simulink library "FIBlockLib"  (R2021a)
settings: Solver=VariableStepAuto  StartTime=0.0  StopTime=10.0  RelTol=1e-3
settings Model: Creator=flata  LastModifiedBy=DELL
settings SolverCC: AlgebraicLoopSolver=TrustRegion
settings DebuggingCC: SFMachineParentedDataDiag=warning

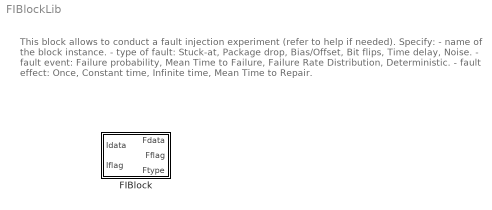
== system FIBlockLib ==
  note: This block allows to conduct a fault injection experiment (refer to help if needed).
      | Specify:
      | - name of the block instance.
      | - type of fault: Stuck-at, Package drop, Bias/Offset, Bit flips, Time delay, Noise.
      | - fault event: Failure probability, Mean Time to Failure, Failure Rate Distribution, Deterministic.
      | - fault effect: Once, Constant time, Infinite time, Mean Time to Repair.
  FIBlock : Subsystem  BlockKeywords=__PRM__SERIALIZED__DATA__:FIBlock,FI Block,FaultInjectionBlock,Fault Injection  TreatAsAtomicUnit=on  mask(Fault Injector Block){FIBlockName=1, FInjEnable=on, FaultType=Stuck-at, FaultValue=1, FaultEvent=Failure probability, EventValue=0.001, FaultEffect=Constant time, EffectValue=1}
      mask prompts: FIBlockName "Number of the FI block instance (e.i. 'name' of the fault injector)"; FInjEnable "Turn on the fault injection for this block"; FaultType "Fault type"; FaultValue "Fault value (bias)"; FaultEvent "Fault injection method"; EventValue "Event value (probability)"; FaultEffect "Fault injection effect"; EffectValue "Effect value (s)"
      mask help:
      | This block allows to conduct a fault injection experiment (refer to help if needed).
      | Specify:
      | - name of the block instance.
      | - type of fault: Stuck-at, Package drop, Bias/Offset, Bit flips, Time delay, Noise.
      | - fault event: Failure probability, Mean Time to Failure, Failure Rate Distribution, Deterministic.
      | - fault effect: Once, Constant time, Infinite time, Mean Time to Repair.
      mask init:
      | % p = Simulink.Mask.get(gcb);
      | % FIBtype = p.getParameter('FaultType');
      | % FIBvalue = p.getParameter('FaultValue');
      | % FaultTypeDesc = p.getDialogControl('FaultTypeDesc');
      | % FIBeffect = p.getParameter('FaultEffect');
      | % FIBeffectval = p.getParameter('EffectValue');
      | % FaultEffectDesc = p.getDialogControl('FaultEffectDesc');
      | % FIBevent = p.getParameter('FaultEvent');
      | % FIBeventval = p.getParameter('EventValue');
      | % FaultEventDesc = p.getDialogControl('FaultEventDesc');
      | % 
      | % if FIBtype.Value == "Stuck-at" || FIBtype.Value == "Time delay"
      | %     FIBvalue.Visible = 'off';
      | % else 
      | %     FIBvalue.Visible = 'on';
      | % end
      | % if FIBeffect.Value == "Infinite time"  || FIBeffect.Value == "Once"
      | %     FIBeffectval.Visible = 'off';
      | % else 
      | %     FIBeffectval.Visible = 'on';
      | % end
      | % 
      | % if FIBtype.Value == "Bias/Offset"
      | %     FIBvalue.Prompt = "Fault value (bias)";
      | %     FaultTypeDesc.Prompt = "The defined positive or negative Bias value is added to the block output.";
      | % elseif FIBtype.Value == "Stuck-at"
      | %     FaultTypeDesc.Prompt = "The block output stays constant, preserving the latest correct value before the error occurrence.";
      | % elseif FIBtype.Value == "Package drop"
      | %     FIBvalue.Prompt = "Fault value";
      | %     FaultTypeDesc.Prompt = "The correct output is replaced by the specified Value, emulating a package drop.";
      | % elseif FIBtype.Value == "Noise"
      | %     FIBvalue.Prompt = "Fault value (boundaries, %)";
      | %     FaultTypeDesc.Prompt = "A random noise value is added. The Boundaries are defined as the percentage of the correct value.";
      | % elseif FIBtype.Value == "Time delay"
      | %     FaultTypeDesc.Prompt = "A delay is introduced into the signal. During the delay the value is zero.";
      | % else
      | %     FIBvalue.Prompt = "Fault value (number of bits)";
      | %     FaultTypeDesc.Prompt = "The defined Number of bits are inverted in the binary representation of the correct value.";
      | % end
      | % 
      | % if FIBevent.Value == "Failure probability"
      | %     FIBeventval.Prompt = "Event value (probability)";
      | %     FaultEventDesc.Prompt = "Errors are injected based on the constant Failure probability for each execution of the block function.";
      | % elseif FIBevent.Value == "Mean Time To Failure"
      | %     FIBeventval.Prompt = "Event value (s)";
      | %     FaultEventDesc.Prompt = "Errors are injected according to the specified MTTF. Normal distribution.";
      | % else FIBeventval.Prompt = "Event value (s)";
      | %     FaultEventDesc.Prompt = "Errors are injected at the specified time";
      | % end
      | % 
      | % if FIBeffect.Value == "Once"
      | %     FaultEffectDesc.Prompt = "An error appears only one time during a simulation.";
      | % elseif FIBeffect.Value == "Constant time"
      | %     FIBeffectval.Prompt = "Effect value (s)";
      | %     FaultEffectDesc.Prompt = "The block produces erroneous output during the specified Time period.";
      | % elseif FIBeffect.Value == "Infinite time"
      | %     FaultEffectDesc.Prompt = "The block produces erroneous output until the end of the simulation.";
      | % elseif FIBeffect.Value == "Mean Time To Repair"
      | %     FIBeffectval.Prompt = "Effect value (s)";
      | %     FaultEffectDesc.Prompt = "Normally distributed MTTR regulates the time of the error effect.";
      | % end
      | % 
      | % FIInit
      | % FIInit
      | % %disp('INIT')
      | FIInit
      mask Help:
      | Failure rate distribution is not supported yet!
      | Bit flips, Time delay, and Noise faults may have some bugs :D
      | In different FIBlock instances, the 'name' of the block in GUI must be different (must be an integer number).
      | 
      | Please refer to a comprehensive article regarding the FIBLock: https://flatag.tech/fiblock.html
      | Please cite as: "Fabarisov, T. et al. "Model-based Fault Injection Experiments for the Safety Analysis of Exoskeleton System." Proceedings of the 30th European Safety and Reliability Conference and the 15th Probabilistic Safety Assessment and Management Conference, 2020."
      | 
      | This block allows to conduct a fault injection experiment.
      | Specify:
      | 1) number of the block instance (e.i. 'name' of the fault injector, name shall be unique).
      | 
      | 2) type of fault:
      | - Stuck-at. The block output stays constant, preserving the latest correct value before the error occurrence.
      | - Package drop. The correct output is replaced by the specified Value, emulating a package drop.
      | - Bias/Offset . The defined positive or negative Bias value is added to the block output.
      | - Noise. A random noise value is added. The Boundaries are defined as the percentage of the correct value.
      | - Time delay. A delay is introduced into the signal. During the delay the value is zero.
      | - Bit flips. The defined Number of bits are inverted in the binary representation of the correct value.
      | 
      | 3) fault event:
      | - Failure probability. Errors are injected based on the constant Failure probability for each execution of the block function.
      | - Mean Time to Failure. Errors are injected according to the specified MTTF. Normal distribution.
      | - Deterministic. Уrrors are injected at specific time step.
      | 
      | 4) fault effect:
      | - Once. An error appears only one time during a simulation.
      | - Constant time. The block produces erroneous output during the specified Time period.
      | - Infinite time. The block produces erroneous output until the end of the simulation.
      | - Mean Time to Repair. Normally distributed MTTR regulates the time of the error effect.
      | 
      | FIBlock also provide, what we call, a chained fault injection.
      | Second output of the FIBlock emits a trigger flag.
      | This output signal could be connected to the second input of the FIBlock.
      | In case of the fault injection, this signal will force trigger fault injectionin second FIBlock.
      | 
      | FIBlock supports a base Workspace variables as input in the GUI parameters.
      | 
      | Made By Tagir Fabarisov, TU Dresden 2020
      mask TypeOptions FaultType: Stuck-at | Package drop | Bias/Offset | Bit flips | Time delay | Noise
      mask Callback FaultType:
      | p = Simulink.Mask.get(gcb);
      | FIBtype = p.getParameter('FaultType');
      | FIBvalue = p.getParameter('FaultValue');
      | FaultTypeDesc = p.getDialogControl('FaultTypeDesc');
      | 
      | if FIBtype.Value == "Stuck-at" || FIBtype.Value == "Time delay"
      |     FIBvalue.Visible = 'off';
      | else
      |     FIBvalue.Visible = 'on';
      | end
      | 
      | if FIBtype.Value == "Bias/Offset"
      |     FIBvalue.Prompt = "Fault value (bias)";
      |     FaultTypeDesc.Prompt = "The defined positive or negative Bias value is added to the block output.";
      | elseif FIBtype.Value == "Stuck-at"
      |     FaultTypeDesc.Prompt = "The block output stays constant, preserving the latest correct value before the error occurrence.";
      | elseif FIBtype.Value == "Package drop"
      |     FIBvalue.Prompt = "Fault value";
      |     FaultTypeDesc.Prompt = "The correct output is replaced by the specified Value, emulating a package drop.";
      | elseif FIBtype.Value == "Noise"
      |     FIBvalue.Prompt = "Fault value (boundaries, %)";
      |     FaultTypeDesc.Prompt = "A random noise value is added. The Boundaries are defined as the percentage of the correct value.";
      | elseif FIBtype.Value == "Time delay"
      |     FaultTypeDesc.Prompt = "A delay is introduced into the signal. During the delay the value is zero.";
      | else
      |     FIBvalue.Prompt = "Fault value (number of bits)";
      |     FaultTypeDesc.Prompt = "The defined Number of bits are inverted in the binary representation of the correct value.";
      | end
      mask TypeOptions FaultEvent: Failure probability | Mean Time To Failure | Deterministic
      mask Callback FaultEvent:
      | p = Simulink.Mask.get(gcb);
      | FIBevent = p.getParameter('FaultEvent');
      | FIBeventval = p.getParameter('EventValue');
      | FaultEventDesc = p.getDialogControl('FaultEventDesc');
      | 
      | if FIBevent.Value == "Failure probability"
      |     FIBeventval.Prompt = "Event value (probability)";
      |     FaultEventDesc.Prompt = "Errors are injected based on the constant Failure probability for each execution of the block function.";
      | elseif FIBevent.Value == "Mean Time To Failure"
      |     FIBeventval.Prompt = "Event value (s)";
      |     FaultEventDesc.Prompt = "Errors are injected according to the specified MTTF. Normal distribution.";
      | else FIBeventval.Prompt = "Event value (s)";
      |     FaultEventDesc.Prompt = "Errors are injected at the specified time";
      | end
      mask TypeOptions FaultEffect: Once | Constant time | Infinite time | Mean Time To Repair
      mask Callback FaultEffect:
      | p = Simulink.Mask.get(gcb);
      | 
      | FIBeffect = p.getParameter('FaultEffect');
      | FIBeffectval = p.getParameter('EffectValue');
      | FaultEffectDesc = p.getDialogControl('FaultEffectDesc');
      | 
      | 
      | if FIBeffect.Value == "Infinite time" || FIBeffect.Value == "Once"
      |  FIBeffectval.Visible = 'off';
      | else
      |  FIBeffectval.Visible = 'on';
      | end
      | 
      | 
      | if FIBeffect.Value == "Once"
      |  FaultEffectDesc.Prompt = "An error appears only one time during a simulation.";
      | elseif FIBeffect.Value == "Constant time"
      |  FIBeffectval.Prompt = "Effect value (s)";
      |  FaultEffectDesc.Prompt = "The block produces erroneous output during the specified Time period.";
      | elseif FIBeffect.Value == "Infinite time"
      |  FaultEffectDesc.Prompt = "The block produces erroneous output until the end of the simulation.";
      | elseif FIBeffect.Value == "Mean Time To Repair"
      |  FIBeffectval.Prompt = "Effect value (s)";
      |  FaultEffectDesc.Prompt = "Normally distributed MTTR regulates the time of the error effect.";
      | end
      mask DialogControl FInjEnable Tooltip: If ticked, then this FIBlock will inject faults
      mask DialogControl Container8 Prompt: Fault type
      mask DialogControl FaultType Tooltip: Specify a type of fault that will be injected
      mask DialogControl FaultTypeDesc Prompt: The block output stays constant, preserving the latest correct value before the error occurrence.
      mask DialogControl Container3 Prompt: Fault injection method
      mask DialogControl Container6 Prompt: Event
      mask DialogControl FaultEvent Tooltip: Specify when fault will be injected
      mask DialogControl FaultEventDesc Prompt: Errors are injected based on the constant Failure probability for each execution of the block function.
      mask DialogControl Container7 Prompt: Effect
      mask DialogControl FaultEffect Tooltip: Specify how long fault will be injected
      mask DialogControl FaultEffectDesc Prompt: The block produces erroneous output during the specified Time period.
      mask Display:
      | warning off;
      | color('red');
      | a = FaultType;
      | if a == "Sensor: Stuck-at fault"
      |     color('black');
      |     x = linspace(-pi,pi);
      |     y = sin(x);
      |     plot(x,y);
      |     color('red');
      |     disp('        ↯');
      |     x = [-0.7 2];
      |     y = [-0.7 -0.7];
      |     plot(x,y);
      | elseif a == "Network: Package drop"
      |     color('black');
      |     x = linspace(-pi,pi);
      |     y = sin(x);
      |     plot(x,y);
      |     color('red');
      |     disp('        ↯');
      |     x = [-0.7 -0.7];
      |     y = [-0.7 0];
      |     plot(x,y);
      |     x = [-0.7 1];
      |     y = [0 0];
      |     plot(x,y);
      | elseif a == "Sensor: Offset"
      |     color('black');
      |     x1 = linspace(-pi,pi);
      |     y1 = sin(x1)-0.5;
      |     plot(x1,y1);
      |     color('red');
      |     disp('        ↯');
      |     x2 = linspace(0,pi);
      |     y2 = sin(x2);
      |     plot(x2,y2);
      |     x = [0 0];
      |     y = [-0.5 0];
      |     plot(x,y);
      | elseif a == "Hardware: Bit flips"
      |     color('black');
      |     disp('10101010');
      |     color('red');
      |     disp('    0↯');
      | elseif a == "Network: Time delay"
      |     color('black');
      |     x1 = linspace(-pi,pi);
      |     y1 = sin(x1);
      |     plot(x1,y1);
      |     color('red');
      |     disp('        ↯');
      |     x2 = linspace(0,pi);
      |     y2 = sin(x2-0.5);
      |     plot(x2,y2);
      |     x = [0 -0.4];
      |     y = [-0.5 -0.5];
      |     plot(x,y);
      | elseif a == "Sensor: Noise"
      |     color('black');
      |     x1 = linspace(-pi,pi);
      |     y1 = sin(x1);
      |     plot(x1,y1);
      |     color('red');
      |     disp('        ↯');
      |     x = linspace(-pi/8,pi/8,10);
      |     y = sin(x);
      |     for yc = 1:length(y)
      |         d = randi([-2,2])/5;
      |         y(yc) = y(yc) + d;
      |     end
      |     plot(x,y);
      | else
      |     color('red');
      |     disp('Set up Fault Injector!');
      | %Bit flips
      | %Time delay
      | %Noise
      | end
      | warning on;

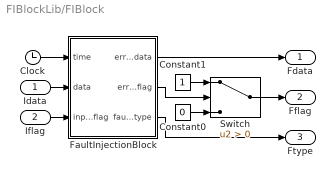
== system FIBlockLib/FIBlock ==
  Idata : Inport
  Iflag : Inport  Port=2
  Clock : Clock
  Constant0 : Constant  Value=0
  Constant1 : Constant
  FaultInjectionBlock : MATLAB Function  TreatAsAtomicUnit=on  SystemSampleTime=0.005
  Switch : Switch  Criteria=u2 > Threshold
  Fdata : Outport
  Fflag : Outport  Port=2
  Ftype : Outport  Port=3
  wires:
  Idata/1 -> FaultInjectionBlock/2(data)
  Clock/1 -> FaultInjectionBlock/1(time)
  FaultInjectionBlock/1(error_data) -> Fdata/1
  Iflag/1 -> FaultInjectionBlock/3(input_flag)
  Constant0/1 -> Switch/3
  Constant1/1 -> Switch/1
  FaultInjectionBlock/2(error_flag) -> Switch/2
  Switch/1 -> Fflag/1
  FaultInjectionBlock/3(fault_type) -> Ftype/1

== matlab function FIBlockLib/FIBlock/FaultInjectionBlock ==
  data: time input; error_data output; data input; input_flag input; FIBlockName parameter; error_flag output; fault_type output
function [error_data, error_flag, fault_type] = fcn(time, data, input_flag, FIBlockName)
coder.extrinsic('wrapper');
d = data;
t = time;
n = num2str(FIBlockName);
f = input_flag;
error_data = coder.nullcopy(zeros(size(d)));
error_flag = 0;
fault_type = 0;
[error_data, error_flag, fault_type] = wrapper(d, t, n, f);
end
